simulink model "ex_3s1"  (R2018b)
settings: Solver=ode5  StartTime=0.0  StopTime=10.0  FixedStep=0.001  RelTol=1e-3
libraries: discretizing x1
settings Model: Creator=lenovo  LastModifiedBy=QJ-
settings DebuggingCC: LibraryContextMissingDiagnostic=none
settings SFSimCC: SimUseLocalCustomCode=off
settings RTWCC: RTWUseLocalCustomCode=off

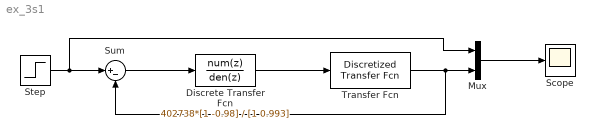
== system ex_3s1 ==
  Discrete Transfer Fcn : DiscreteTransferFcn  Numerator=402738*[1 -0.98]  Denominator=[1 0.993]  SampleTime=0.001
  Mux : Mux  Inputs=2
  Scope : Scope
  Step : Step  SampleTime=0.001  mask(DiscretizedSource){}
      mask init:
      | %zoh
  Sum : Sum  Inputs=|+-
  Transfer Fcn : discretizing/Discretized Transfer Fcn  Numerator=[5]  Denominator=[1 20 0]  AbsTol=auto  SampleTime=0.001  method=zoh  Wc=0
  wires:
  Discrete Transfer Fcn/1 -> Transfer Fcn/1
  Sum/1 -> Discrete Transfer Fcn/1
  Step/1 -> Mux/1, Sum/1
  Transfer Fcn/1 -> Sum/2, Mux/2
  Mux/1 -> Scope/1
